simulink library "RoboCar"  (R2023a)
settings: Solver=VariableStepAuto  StartTime=0.0  StopTime=10.0  RelTol=1e-3
settings Model: Creator=Franz  LastModifiedBy=Franz

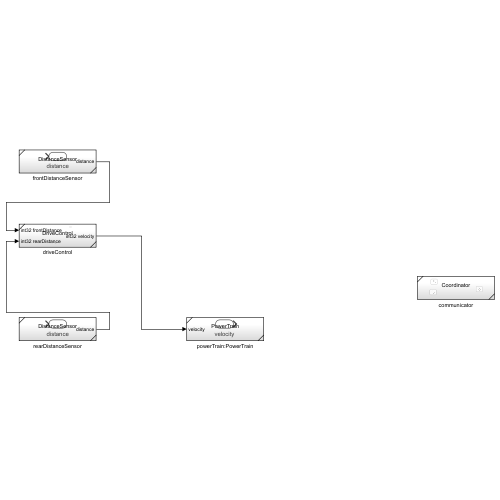
[thumbnail: Simulink's stored preview of the top-level diagram]
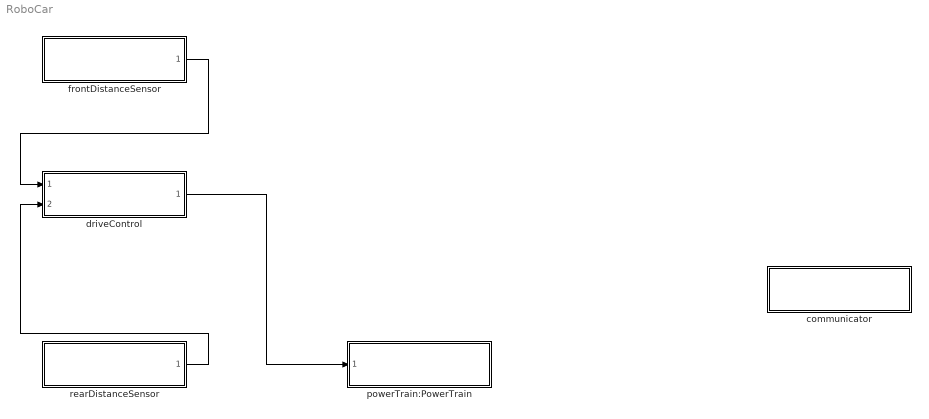
== system RoboCar ==
  communicator : Subsystem  ReferencedSubsystem=Coordinator
  driveControl : Subsystem  ReferencedSubsystem=DriveControl
  frontDistanceSensor : Subsystem  ReferencedSubsystem=DistanceSensor
  powerTrain:PowerTrain : Subsystem  ReferencedSubsystem=PowerTrain
  rearDistanceSensor : Subsystem  ReferencedSubsystem=DistanceSensor
  wires:
  driveControl/1 -> powerTrain:PowerTrain/1
  frontDistanceSensor/1 -> driveControl/1
  rearDistanceSensor/1 -> driveControl/2
